simulink model "ProdSys_MakeToOrderPUSH_optionalWIPCap"  (R2015a)
settings: Solver=ode45  SolverMode=SingleTasking  StartTime=0.0  StopTime=10.0  RelTol=1e-3
undefined symbols (not defined in the file or in its folder): se_randomizeseeds
libraries: simeventslib x6, simulink x1
(part 2 of 2)

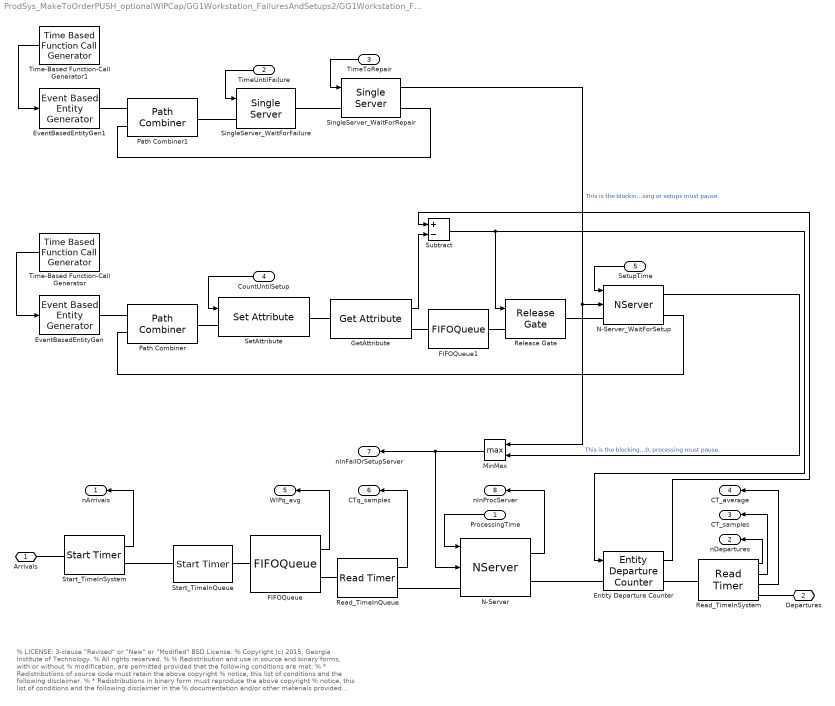
== system ProdSys_MakeToOrderPUSH_optionalWIPCap/GG1Workstation_FailuresAndSetups2/GG1Workstation_FailuresAndSetups ==
  note: % LICENSE: 3-clause "Revised" or "New" or "Modified" BSD License.
      | % Copyright (c) 2015, Georgia Institute of Technology.
      | % All rights reserved.
      | %
      | % Redistribution and use in source and binary forms, with or without
      | % modification, are permitted provided that the following conditions are met:
      | % * Redistributions of source code must retain the above copyright
      | % notice, this list of conditions and the following disclaimer.
      | % * Redistributions in binary form must reproduce the above copyright
      | % notice, this list of conditions and the following disclaimer in the
      | % documentation and/or other materials provided with the distribution.
      | % * Neither the name of the Georgia Institute of Technology nor the
      | % names of its contributors may be used to endorse or promote products
      | % derived from this software without specific prior written permission.
      | %
      | % THIS SOFTWARE IS PROVIDED BY THE COPYRIGHT HOLDERS AND CONTRIBUTORS "AS IS" AND
      | % ANY EXPRESS OR IMPLIED WARRANTIES, INCLUDING, BUT NOT LIMITED TO, THE IMPLIED
      | % WARRANTIES OF MERCHANTABILITY AND FITNESS FOR A PARTICULAR PURPOSE ARE
      | % DISCLAIMED. IN NO EVENT SHALL THE GEORGIA INSTITUTE OF TECHNOLOGY BE LIABLE FOR
      | % ANY DIRECT, INDIRECT, INCIDENTAL, SPECIAL, EXEMPLARY, OR CONSEQUENTIAL DAMAGES
      | % (INCLUDING, BUT NOT LIMITED TO, PROCUREMENT OF SUBSTITUTE GOODS OR SERVICES;
      | % LOSS OF USE, DATA, OR PROFITS; OR BUSINESS INTERRUPTION) HOWEVER CAUSED AND
      | % ON ANY THEORY OF LIABILITY, WHETHER IN CONTRACT, STRICT LIABILITY, OR TORT
      | % (INCLUDING NEGLIGENCE OR OTHERWISE) ARISING IN ANY WAY OUT OF THE USE OF THIS
      | % SOFTWARE, EVEN IF ADVISED OF THE POSSIBILITY OF SUCH DAMAGE.
  ProcessingTime : Inport
  TimeUntilFailure : Inport  Port=2
  TimeToRepair : Inport  Port=3
  CountUntilSetup : Inport  Port=4
  SetupTime : Inport  Port=5
  Entity Departure Counter : EntityDepartureCounter  NumberDepartedToSignal=on  NumberDepartedToAttribute=off  CounterResetTypeOption=Trigger from port tr
  EventBasedEntityGen : EventBasedEntityGenerator  GenerateEntitiesUpon=Function call from port fcn
  EventBasedEntityGen1 : EventBasedEntityGenerator  GenerateEntitiesUpon=Function call from port fcn
  FIFOQueue : FIFOQueue  Capacity=Capacity  StatAverageQueueLength=on
      settings: OutputPortMap=o3
  FIFOQueue1 : FIFOQueue  Capacity=Inf
  GetAttribute : GetAttribute  AttributeName=CountUntilSetup  EvaluatedDefaultAttributeValue={ []}
      settings: OutputPortMap=o1
  MinMax : MinMax  Function=max  Inputs=2
  N-Server : NServer  NumberOfServers=1  ServiceTimeFrom=Signal port t  AllowServiceControl=on  BlockWhileSignalOn=on  StatNumberInBlock=on
      settings: InputPortMap=u0,u1  OutputPortMap=o1
  N-Server_WaitForSetup : NServer  NumberOfServers=1  ServiceTimeFrom=Signal port t  AllowServiceControl=on  BlockWhileSignalOn=on  StatNumberInBlock=on
      settings: InputPortMap=u0,u1  OutputPortMap=o1
  Path Combiner : PathCombiner  NumberInputPorts=2
  Path Combiner1 : PathCombiner  NumberInputPorts=2
  Read_TimeInQueue : ReadTimer  TimerTag=TimeInQueue  StatTimeElapsed=on
      settings: OutputPortMap=o2
  Read_TimeInSystem : ReadTimer  TimerTag=TimeInSystem  StatNumberDeparted=on  StatTimeElapsed=on  StatAverageTimeElapsed=on
      settings: OutputPortMap=o0,o2,o3
  Release Gate : ReleaseGate  OpenGateUpon=Trigger from port tr
  SetAttribute : SetAttribute  AttributeName=CountUntilSetup  AttributeFrom=Signal port  EvaluatedAttributeValue={ []}
  SingleServer_WaitForFailure : SingleServer  ServiceTimeFrom=Signal port t  AttributeName=TimeUntilFailure
  SingleServer_WaitForRepair : SingleServer  ServiceTimeFrom=Signal port t  AttributeName=TimeToRepair  StatNumberInBlock=on
      settings: OutputPortMap=o1
  Start_TimeInQueue : StartTimer  TimerTag=TimeInQueue  TimerStartedOption=Restart
  Start_TimeInSystem : StartTimer  TimerTag=TimeInSystem  TimerStartedOption=Restart  StatNumberDeparted=on
  Subtract : Sum  Inputs=+-
  Time-Based Function-Call Generator : TimeBasedFunctionCallGenerator  EventGenerationMode=Only at simulation start
  Time-Based Function-Call Generator1 : TimeBasedFunctionCallGenerator  EventGenerationMode=Only at simulation start
  Arrivals : PMIOPort  Port=1  Side=Left
  Departures : PMIOPort  Port=2  Side=Right
  nArrivals : Outport
  nDepartures : Outport  Port=2
  CT_samples : Outport  Port=3
  CT_average : Outport  Port=4
  WIPq_avg : Outport  Port=5
  CTq_samples : Outport  Port=6
  nInFailOrSetupServer : Outport  Port=7
  nInProcServer : Outport  Port=8
  wires:
  MinMax/1 -> N-Server/2, nInFailOrSetupServer/1
  N-Server_WaitForSetup/1 -> MinMax/2  "This is the blocking signal from setups.  When >0, processing must pause."
  SingleServer_WaitForRepair/1 -> N-Server_WaitForSetup/2, MinMax/1  "This is the blocking signal from failures. When >0, processing or setups must pause."
  TimeUntilFailure/1 -> SingleServer_WaitForFailure/1
  TimeToRepair/1 -> SingleServer_WaitForRepair/1
  Time-Based Function-Call Generator1/1 -> EventBasedEntityGen1/1
  SetupTime/1 -> N-Server_WaitForSetup/1
  N-Server/1 -> nInProcServer/1
  Entity Departure Counter/1 -> Subtract/1
  GetAttribute/1 -> Subtract/2
  Subtract/1 -> Entity Departure Counter/1, Release Gate/1
  CountUntilSetup/1 -> SetAttribute/1
  Time-Based Function-Call Generator/1 -> EventBasedEntityGen/1
  Read_TimeInSystem/3 -> CT_average/1
  ProcessingTime/1 -> N-Server/1
  Read_TimeInSystem/1 -> nDepartures/1
  Start_TimeInSystem/1 -> nArrivals/1
  FIFOQueue/1 -> WIPq_avg/1
  Read_TimeInQueue/1 -> CTq_samples/1
  Read_TimeInSystem/2 -> CT_samples/1
  connections:
  Path Combiner1/RConn1 -- SingleServer_WaitForFailure/LConn1
  EventBasedEntityGen1/RConn1 -- Path Combiner1/LConn1
  SingleServer_WaitForRepair/LConn1 -- SingleServer_WaitForFailure/RConn1
  Path Combiner1/LConn2 -- SingleServer_WaitForRepair/RConn1
  SetAttribute/RConn1 -- GetAttribute/LConn1
  FIFOQueue1/RConn1 -- Release Gate/LConn1
  N-Server_WaitForSetup/LConn1 -- Release Gate/RConn1
  FIFOQueue1/LConn1 -- GetAttribute/RConn1
  Entity Departure Counter/RConn1 -- Read_TimeInSystem/LConn1
  N-Server/RConn1 -- Entity Departure Counter/LConn1
  Path Combiner/LConn2 -- N-Server_WaitForSetup/RConn1
  EventBasedEntityGen/RConn1 -- Path Combiner/LConn1
  Path Combiner/RConn1 -- SetAttribute/LConn1
  Start_TimeInQueue/RConn1 -- FIFOQueue/LConn1
  Read_TimeInQueue/RConn1 -- N-Server/LConn1
  Read_TimeInSystem/RConn1 -- Departures/RConn1
  Start_TimeInSystem/RConn1 -- Start_TimeInQueue/LConn1
  FIFOQueue/RConn1 -- Read_TimeInQueue/LConn1
  Arrivals/RConn1 -- Start_TimeInSystem/LConn1

== system ProdSys_MakeToOrderPUSH_optionalWIPCap/GG1Workstation_FailuresAndSetups3/ComputeTH ==
  CurrentTime : Inport
  nDepartures : Inport  Port=2
  Derivative : Derivative
  Divide1 : Product  Inputs=/*
  Event to Timed Signal1 : EventToTimedSignal
  TH_average : Outport
  TH_samples : Outport  Port=2
  wires:
  nDepartures/1 -> Event to Timed Signal1/1
  Derivative/1 -> TH_samples/1
  Divide1/1 -> TH_average/1
  Event to Timed Signal1/1 -> Divide1/2, Derivative/1
  CurrentTime/1 -> Divide1/1

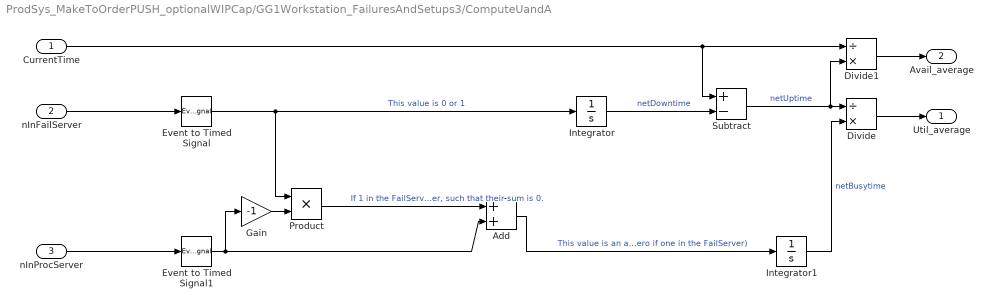
== system ProdSys_MakeToOrderPUSH_optionalWIPCap/GG1Workstation_FailuresAndSetups3/ComputeUandA ==
  CurrentTime : Inport
  nInFailServer : Inport  Port=2
  nInProcServer : Inport  Port=3
  Add : Sum
  Divide : Product  Inputs=/*
  Divide1 : Product  Inputs=/*
  Event to Timed Signal : EventToTimedSignal
  Event to Timed Signal1 : EventToTimedSignal
  Gain : Gain  Gain=-1
  Integrator : Integrator
  Integrator1 : Integrator
  Product : Product
  Subtract : Sum  Inputs=+-
  Util_average : Outport
  Avail_average : Outport  Port=2
  wires:
  Divide1/1 -> Avail_average/1
  Event to Timed Signal1/1 -> Gain/1, Add/2
  Add/1 -> Integrator1/1  "This value is an adjusted number in the ProcServer (zero if one in the FailServer)"
  Product/1 -> Add/1  "If 1 in the FailServer, then this value should be negative the number in the ProcServer, such that their sum is 0."
  Gain/1 -> Product/2
  Integrator1/1 -> Divide/2  "netBusytime"
  Subtract/1 -> Divide1/2, Divide/1  "netUptime"
  Divide/1 -> Util_average/1
  CurrentTime/1 -> Divide1/1, Subtract/1
  Integrator/1 -> Subtract/2  "netDowntime"
  nInProcServer/1 -> Event to Timed Signal1/1
  nInFailServer/1 -> Event to Timed Signal/1
  Event to Timed Signal/1 -> Product/1, Integrator/1  "This value is 0 or 1"

== system ProdSys_MakeToOrderPUSH_optionalWIPCap/GG1Workstation_FailuresAndSetups3/ComputeWIP ==
  nArrivals : Inport
  nDepartures : Inport  Port=2
  CurrentTime : Inport  Port=3
  Divide : Product  Inputs=*/
  Event to Timed Signal : EventToTimedSignal
  Integrator : Integrator
  Subtract : Sum  Inputs=+-
  WIP_samples : Outport
  WIP_average : Outport  Port=2
  wires:
  CurrentTime/1 -> Divide/2
  nDepartures/1 -> Subtract/2
  nArrivals/1 -> Subtract/1
  Integrator/1 -> Divide/1
  Divide/1 -> WIP_average/1
  Event to Timed Signal/1 -> Integrator/1
  Subtract/1 -> Event to Timed Signal/1, WIP_samples/1

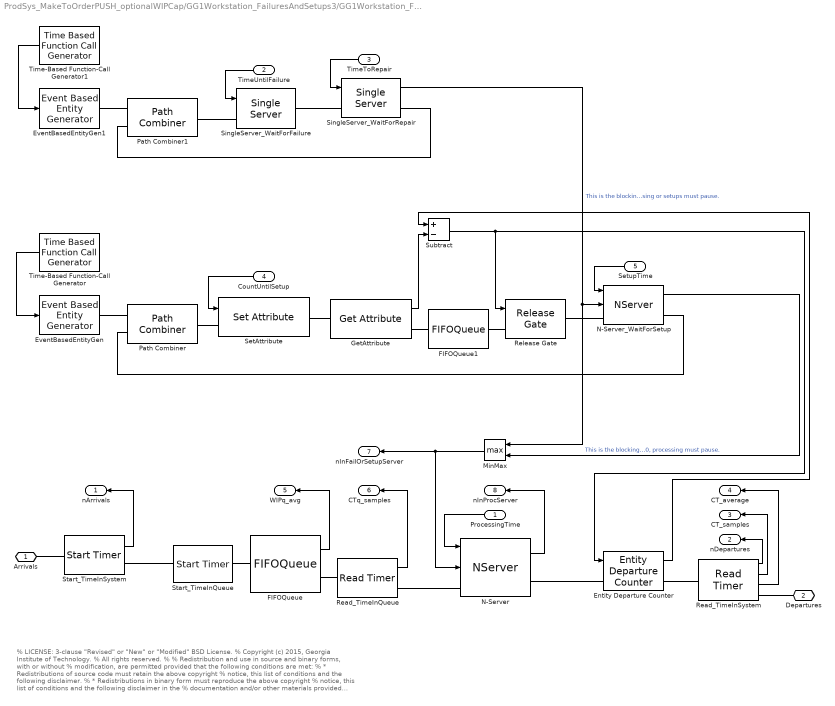
== system ProdSys_MakeToOrderPUSH_optionalWIPCap/GG1Workstation_FailuresAndSetups3/GG1Workstation_FailuresAndSetups ==
  note: % LICENSE: 3-clause "Revised" or "New" or "Modified" BSD License.
      | % Copyright (c) 2015, Georgia Institute of Technology.
      | % All rights reserved.
      | %
      | % Redistribution and use in source and binary forms, with or without
      | % modification, are permitted provided that the following conditions are met:
      | % * Redistributions of source code must retain the above copyright
      | % notice, this list of conditions and the following disclaimer.
      | % * Redistributions in binary form must reproduce the above copyright
      | % notice, this list of conditions and the following disclaimer in the
      | % documentation and/or other materials provided with the distribution.
      | % * Neither the name of the Georgia Institute of Technology nor the
      | % names of its contributors may be used to endorse or promote products
      | % derived from this software without specific prior written permission.
      | %
      | % THIS SOFTWARE IS PROVIDED BY THE COPYRIGHT HOLDERS AND CONTRIBUTORS "AS IS" AND
      | % ANY EXPRESS OR IMPLIED WARRANTIES, INCLUDING, BUT NOT LIMITED TO, THE IMPLIED
      | % WARRANTIES OF MERCHANTABILITY AND FITNESS FOR A PARTICULAR PURPOSE ARE
      | % DISCLAIMED. IN NO EVENT SHALL THE GEORGIA INSTITUTE OF TECHNOLOGY BE LIABLE FOR
      | % ANY DIRECT, INDIRECT, INCIDENTAL, SPECIAL, EXEMPLARY, OR CONSEQUENTIAL DAMAGES
      | % (INCLUDING, BUT NOT LIMITED TO, PROCUREMENT OF SUBSTITUTE GOODS OR SERVICES;
      | % LOSS OF USE, DATA, OR PROFITS; OR BUSINESS INTERRUPTION) HOWEVER CAUSED AND
      | % ON ANY THEORY OF LIABILITY, WHETHER IN CONTRACT, STRICT LIABILITY, OR TORT
      | % (INCLUDING NEGLIGENCE OR OTHERWISE) ARISING IN ANY WAY OUT OF THE USE OF THIS
      | % SOFTWARE, EVEN IF ADVISED OF THE POSSIBILITY OF SUCH DAMAGE.
  ProcessingTime : Inport
  TimeUntilFailure : Inport  Port=2
  TimeToRepair : Inport  Port=3
  CountUntilSetup : Inport  Port=4
  SetupTime : Inport  Port=5
  Entity Departure Counter : EntityDepartureCounter  NumberDepartedToSignal=on  NumberDepartedToAttribute=off  CounterResetTypeOption=Trigger from port tr
  EventBasedEntityGen : EventBasedEntityGenerator  GenerateEntitiesUpon=Function call from port fcn
  EventBasedEntityGen1 : EventBasedEntityGenerator  GenerateEntitiesUpon=Function call from port fcn
  FIFOQueue : FIFOQueue  Capacity=Capacity  StatAverageQueueLength=on
      settings: OutputPortMap=o3
  FIFOQueue1 : FIFOQueue  Capacity=Inf
  GetAttribute : GetAttribute  AttributeName=CountUntilSetup  EvaluatedDefaultAttributeValue={ []}
      settings: OutputPortMap=o1
  MinMax : MinMax  Function=max  Inputs=2
  N-Server : NServer  NumberOfServers=1  ServiceTimeFrom=Signal port t  AllowServiceControl=on  BlockWhileSignalOn=on  StatNumberInBlock=on
      settings: InputPortMap=u0,u1  OutputPortMap=o1
  N-Server_WaitForSetup : NServer  NumberOfServers=1  ServiceTimeFrom=Signal port t  AllowServiceControl=on  BlockWhileSignalOn=on  StatNumberInBlock=on
      settings: InputPortMap=u0,u1  OutputPortMap=o1
  Path Combiner : PathCombiner  NumberInputPorts=2
  Path Combiner1 : PathCombiner  NumberInputPorts=2
  Read_TimeInQueue : ReadTimer  TimerTag=TimeInQueue  StatTimeElapsed=on
      settings: OutputPortMap=o2
  Read_TimeInSystem : ReadTimer  TimerTag=TimeInSystem  StatNumberDeparted=on  StatTimeElapsed=on  StatAverageTimeElapsed=on
      settings: OutputPortMap=o0,o2,o3
  Release Gate : ReleaseGate  OpenGateUpon=Trigger from port tr
  SetAttribute : SetAttribute  AttributeName=CountUntilSetup  AttributeFrom=Signal port  EvaluatedAttributeValue={ []}
  SingleServer_WaitForFailure : SingleServer  ServiceTimeFrom=Signal port t  AttributeName=TimeUntilFailure
  SingleServer_WaitForRepair : SingleServer  ServiceTimeFrom=Signal port t  AttributeName=TimeToRepair  StatNumberInBlock=on
      settings: OutputPortMap=o1
  Start_TimeInQueue : StartTimer  TimerTag=TimeInQueue  TimerStartedOption=Restart
  Start_TimeInSystem : StartTimer  TimerTag=TimeInSystem  TimerStartedOption=Restart  StatNumberDeparted=on
  Subtract : Sum  Inputs=+-
  Time-Based Function-Call Generator : TimeBasedFunctionCallGenerator  EventGenerationMode=Only at simulation start
  Time-Based Function-Call Generator1 : TimeBasedFunctionCallGenerator  EventGenerationMode=Only at simulation start
  Arrivals : PMIOPort  Port=1  Side=Left
  Departures : PMIOPort  Port=2  Side=Right
  nArrivals : Outport
  nDepartures : Outport  Port=2
  CT_samples : Outport  Port=3
  CT_average : Outport  Port=4
  WIPq_avg : Outport  Port=5
  CTq_samples : Outport  Port=6
  nInFailOrSetupServer : Outport  Port=7
  nInProcServer : Outport  Port=8
  wires:
  MinMax/1 -> N-Server/2, nInFailOrSetupServer/1
  N-Server_WaitForSetup/1 -> MinMax/2  "This is the blocking signal from setups.  When >0, processing must pause."
  SingleServer_WaitForRepair/1 -> N-Server_WaitForSetup/2, MinMax/1  "This is the blocking signal from failures. When >0, processing or setups must pause."
  TimeUntilFailure/1 -> SingleServer_WaitForFailure/1
  TimeToRepair/1 -> SingleServer_WaitForRepair/1
  Time-Based Function-Call Generator1/1 -> EventBasedEntityGen1/1
  SetupTime/1 -> N-Server_WaitForSetup/1
  N-Server/1 -> nInProcServer/1
  Entity Departure Counter/1 -> Subtract/1
  GetAttribute/1 -> Subtract/2
  Subtract/1 -> Entity Departure Counter/1, Release Gate/1
  CountUntilSetup/1 -> SetAttribute/1
  Time-Based Function-Call Generator/1 -> EventBasedEntityGen/1
  Read_TimeInSystem/3 -> CT_average/1
  ProcessingTime/1 -> N-Server/1
  Read_TimeInSystem/1 -> nDepartures/1
  Start_TimeInSystem/1 -> nArrivals/1
  FIFOQueue/1 -> WIPq_avg/1
  Read_TimeInQueue/1 -> CTq_samples/1
  Read_TimeInSystem/2 -> CT_samples/1
  connections:
  Path Combiner1/RConn1 -- SingleServer_WaitForFailure/LConn1
  EventBasedEntityGen1/RConn1 -- Path Combiner1/LConn1
  SingleServer_WaitForRepair/LConn1 -- SingleServer_WaitForFailure/RConn1
  Path Combiner1/LConn2 -- SingleServer_WaitForRepair/RConn1
  SetAttribute/RConn1 -- GetAttribute/LConn1
  FIFOQueue1/RConn1 -- Release Gate/LConn1
  N-Server_WaitForSetup/LConn1 -- Release Gate/RConn1
  FIFOQueue1/LConn1 -- GetAttribute/RConn1
  Entity Departure Counter/RConn1 -- Read_TimeInSystem/LConn1
  N-Server/RConn1 -- Entity Departure Counter/LConn1
  Path Combiner/LConn2 -- N-Server_WaitForSetup/RConn1
  EventBasedEntityGen/RConn1 -- Path Combiner/LConn1
  Path Combiner/RConn1 -- SetAttribute/LConn1
  Start_TimeInQueue/RConn1 -- FIFOQueue/LConn1
  Read_TimeInQueue/RConn1 -- N-Server/LConn1
  Read_TimeInSystem/RConn1 -- Departures/RConn1
  Start_TimeInSystem/RConn1 -- Start_TimeInQueue/LConn1
  FIFOQueue/RConn1 -- Read_TimeInQueue/LConn1
  Arrivals/RConn1 -- Start_TimeInSystem/LConn1

== system ProdSys_MakeToOrderPUSH_optionalWIPCap/GG1Workstation_FailuresAndSetups4/ComputeTH ==
  CurrentTime : Inport
  nDepartures : Inport  Port=2
  Derivative : Derivative
  Divide1 : Product  Inputs=/*
  Event to Timed Signal1 : EventToTimedSignal
  TH_average : Outport
  TH_samples : Outport  Port=2
  wires:
  nDepartures/1 -> Event to Timed Signal1/1
  Derivative/1 -> TH_samples/1
  Divide1/1 -> TH_average/1
  Event to Timed Signal1/1 -> Divide1/2, Derivative/1
  CurrentTime/1 -> Divide1/1

== system ProdSys_MakeToOrderPUSH_optionalWIPCap/GG1Workstation_FailuresAndSetups4/ComputeUandA ==
  CurrentTime : Inport
  nInFailServer : Inport  Port=2
  nInProcServer : Inport  Port=3
  Add : Sum
  Divide : Product  Inputs=/*
  Divide1 : Product  Inputs=/*
  Event to Timed Signal : EventToTimedSignal
  Event to Timed Signal1 : EventToTimedSignal
  Gain : Gain  Gain=-1
  Integrator : Integrator
  Integrator1 : Integrator
  Product : Product
  Subtract : Sum  Inputs=+-
  Util_average : Outport
  Avail_average : Outport  Port=2
  wires:
  Divide1/1 -> Avail_average/1
  Event to Timed Signal1/1 -> Gain/1, Add/2
  Add/1 -> Integrator1/1  "This value is an adjusted number in the ProcServer (zero if one in the FailServer)"
  Product/1 -> Add/1  "If 1 in the FailServer, then this value should be negative the number in the ProcServer, such that their sum is 0."
  Gain/1 -> Product/2
  Integrator1/1 -> Divide/2  "netBusytime"
  Subtract/1 -> Divide1/2, Divide/1  "netUptime"
  Divide/1 -> Util_average/1
  CurrentTime/1 -> Divide1/1, Subtract/1
  Integrator/1 -> Subtract/2  "netDowntime"
  nInProcServer/1 -> Event to Timed Signal1/1
  nInFailServer/1 -> Event to Timed Signal/1
  Event to Timed Signal/1 -> Product/1, Integrator/1  "This value is 0 or 1"

== system ProdSys_MakeToOrderPUSH_optionalWIPCap/GG1Workstation_FailuresAndSetups4/ComputeWIP ==
  nArrivals : Inport
  nDepartures : Inport  Port=2
  CurrentTime : Inport  Port=3
  Divide : Product  Inputs=*/
  Event to Timed Signal : EventToTimedSignal
  Integrator : Integrator
  Subtract : Sum  Inputs=+-
  WIP_samples : Outport
  WIP_average : Outport  Port=2
  wires:
  CurrentTime/1 -> Divide/2
  nDepartures/1 -> Subtract/2
  nArrivals/1 -> Subtract/1
  Integrator/1 -> Divide/1
  Divide/1 -> WIP_average/1
  Event to Timed Signal/1 -> Integrator/1
  Subtract/1 -> Event to Timed Signal/1, WIP_samples/1

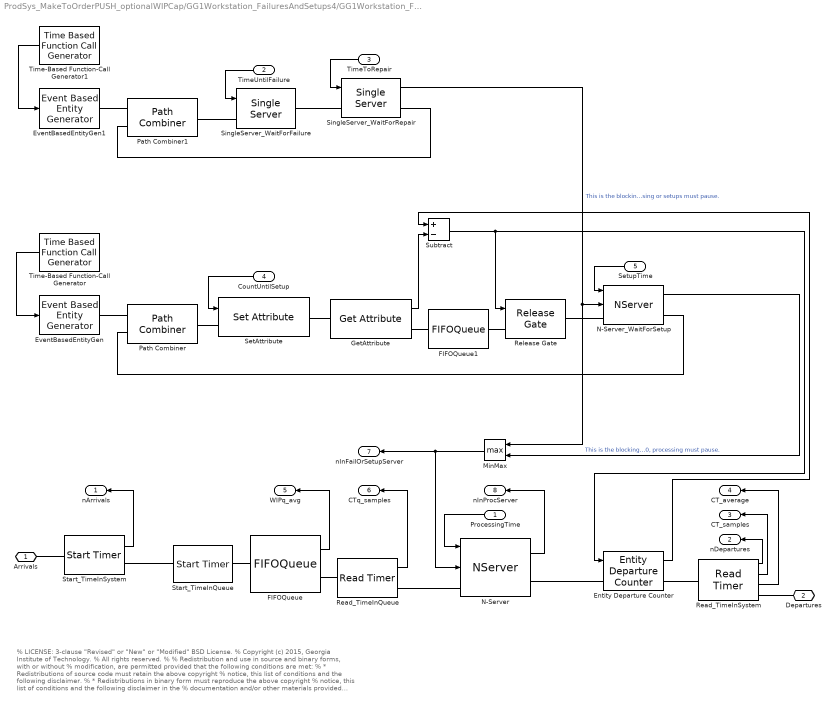
== system ProdSys_MakeToOrderPUSH_optionalWIPCap/GG1Workstation_FailuresAndSetups4/GG1Workstation_FailuresAndSetups ==
  note: % LICENSE: 3-clause "Revised" or "New" or "Modified" BSD License.
      | % Copyright (c) 2015, Georgia Institute of Technology.
      | % All rights reserved.
      | %
      | % Redistribution and use in source and binary forms, with or without
      | % modification, are permitted provided that the following conditions are met:
      | % * Redistributions of source code must retain the above copyright
      | % notice, this list of conditions and the following disclaimer.
      | % * Redistributions in binary form must reproduce the above copyright
      | % notice, this list of conditions and the following disclaimer in the
      | % documentation and/or other materials provided with the distribution.
      | % * Neither the name of the Georgia Institute of Technology nor the
      | % names of its contributors may be used to endorse or promote products
      | % derived from this software without specific prior written permission.
      | %
      | % THIS SOFTWARE IS PROVIDED BY THE COPYRIGHT HOLDERS AND CONTRIBUTORS "AS IS" AND
      | % ANY EXPRESS OR IMPLIED WARRANTIES, INCLUDING, BUT NOT LIMITED TO, THE IMPLIED
      | % WARRANTIES OF MERCHANTABILITY AND FITNESS FOR A PARTICULAR PURPOSE ARE
      | % DISCLAIMED. IN NO EVENT SHALL THE GEORGIA INSTITUTE OF TECHNOLOGY BE LIABLE FOR
      | % ANY DIRECT, INDIRECT, INCIDENTAL, SPECIAL, EXEMPLARY, OR CONSEQUENTIAL DAMAGES
      | % (INCLUDING, BUT NOT LIMITED TO, PROCUREMENT OF SUBSTITUTE GOODS OR SERVICES;
      | % LOSS OF USE, DATA, OR PROFITS; OR BUSINESS INTERRUPTION) HOWEVER CAUSED AND
      | % ON ANY THEORY OF LIABILITY, WHETHER IN CONTRACT, STRICT LIABILITY, OR TORT
      | % (INCLUDING NEGLIGENCE OR OTHERWISE) ARISING IN ANY WAY OUT OF THE USE OF THIS
      | % SOFTWARE, EVEN IF ADVISED OF THE POSSIBILITY OF SUCH DAMAGE.
  ProcessingTime : Inport
  TimeUntilFailure : Inport  Port=2
  TimeToRepair : Inport  Port=3
  CountUntilSetup : Inport  Port=4
  SetupTime : Inport  Port=5
  Entity Departure Counter : EntityDepartureCounter  NumberDepartedToSignal=on  NumberDepartedToAttribute=off  CounterResetTypeOption=Trigger from port tr
  EventBasedEntityGen : EventBasedEntityGenerator  GenerateEntitiesUpon=Function call from port fcn
  EventBasedEntityGen1 : EventBasedEntityGenerator  GenerateEntitiesUpon=Function call from port fcn
  FIFOQueue : FIFOQueue  Capacity=Capacity  StatAverageQueueLength=on
      settings: OutputPortMap=o3
  FIFOQueue1 : FIFOQueue  Capacity=Inf
  GetAttribute : GetAttribute  AttributeName=CountUntilSetup  EvaluatedDefaultAttributeValue={ []}
      settings: OutputPortMap=o1
  MinMax : MinMax  Function=max  Inputs=2
  N-Server : NServer  NumberOfServers=1  ServiceTimeFrom=Signal port t  AllowServiceControl=on  BlockWhileSignalOn=on  StatNumberInBlock=on
      settings: InputPortMap=u0,u1  OutputPortMap=o1
  N-Server_WaitForSetup : NServer  NumberOfServers=1  ServiceTimeFrom=Signal port t  AllowServiceControl=on  BlockWhileSignalOn=on  StatNumberInBlock=on
      settings: InputPortMap=u0,u1  OutputPortMap=o1
  Path Combiner : PathCombiner  NumberInputPorts=2
  Path Combiner1 : PathCombiner  NumberInputPorts=2
  Read_TimeInQueue : ReadTimer  TimerTag=TimeInQueue  StatTimeElapsed=on
      settings: OutputPortMap=o2
  Read_TimeInSystem : ReadTimer  TimerTag=TimeInSystem  StatNumberDeparted=on  StatTimeElapsed=on  StatAverageTimeElapsed=on
      settings: OutputPortMap=o0,o2,o3
  Release Gate : ReleaseGate  OpenGateUpon=Trigger from port tr
  SetAttribute : SetAttribute  AttributeName=CountUntilSetup  AttributeFrom=Signal port  EvaluatedAttributeValue={ []}
  SingleServer_WaitForFailure : SingleServer  ServiceTimeFrom=Signal port t  AttributeName=TimeUntilFailure
  SingleServer_WaitForRepair : SingleServer  ServiceTimeFrom=Signal port t  AttributeName=TimeToRepair  StatNumberInBlock=on
      settings: OutputPortMap=o1
  Start_TimeInQueue : StartTimer  TimerTag=TimeInQueue  TimerStartedOption=Restart
  Start_TimeInSystem : StartTimer  TimerTag=TimeInSystem  TimerStartedOption=Restart  StatNumberDeparted=on
  Subtract : Sum  Inputs=+-
  Time-Based Function-Call Generator : TimeBasedFunctionCallGenerator  EventGenerationMode=Only at simulation start
  Time-Based Function-Call Generator1 : TimeBasedFunctionCallGenerator  EventGenerationMode=Only at simulation start
  Arrivals : PMIOPort  Port=1  Side=Left
  Departures : PMIOPort  Port=2  Side=Right
  nArrivals : Outport
  nDepartures : Outport  Port=2
  CT_samples : Outport  Port=3
  CT_average : Outport  Port=4
  WIPq_avg : Outport  Port=5
  CTq_samples : Outport  Port=6
  nInFailOrSetupServer : Outport  Port=7
  nInProcServer : Outport  Port=8
  wires:
  MinMax/1 -> N-Server/2, nInFailOrSetupServer/1
  N-Server_WaitForSetup/1 -> MinMax/2  "This is the blocking signal from setups.  When >0, processing must pause."
  SingleServer_WaitForRepair/1 -> N-Server_WaitForSetup/2, MinMax/1  "This is the blocking signal from failures. When >0, processing or setups must pause."
  TimeUntilFailure/1 -> SingleServer_WaitForFailure/1
  TimeToRepair/1 -> SingleServer_WaitForRepair/1
  Time-Based Function-Call Generator1/1 -> EventBasedEntityGen1/1
  SetupTime/1 -> N-Server_WaitForSetup/1
  N-Server/1 -> nInProcServer/1
  Entity Departure Counter/1 -> Subtract/1
  GetAttribute/1 -> Subtract/2
  Subtract/1 -> Entity Departure Counter/1, Release Gate/1
  CountUntilSetup/1 -> SetAttribute/1
  Time-Based Function-Call Generator/1 -> EventBasedEntityGen/1
  Read_TimeInSystem/3 -> CT_average/1
  ProcessingTime/1 -> N-Server/1
  Read_TimeInSystem/1 -> nDepartures/1
  Start_TimeInSystem/1 -> nArrivals/1
  FIFOQueue/1 -> WIPq_avg/1
  Read_TimeInQueue/1 -> CTq_samples/1
  Read_TimeInSystem/2 -> CT_samples/1
  connections:
  Path Combiner1/RConn1 -- SingleServer_WaitForFailure/LConn1
  EventBasedEntityGen1/RConn1 -- Path Combiner1/LConn1
  SingleServer_WaitForRepair/LConn1 -- SingleServer_WaitForFailure/RConn1
  Path Combiner1/LConn2 -- SingleServer_WaitForRepair/RConn1
  SetAttribute/RConn1 -- GetAttribute/LConn1
  FIFOQueue1/RConn1 -- Release Gate/LConn1
  N-Server_WaitForSetup/LConn1 -- Release Gate/RConn1
  FIFOQueue1/LConn1 -- GetAttribute/RConn1
  Entity Departure Counter/RConn1 -- Read_TimeInSystem/LConn1
  N-Server/RConn1 -- Entity Departure Counter/LConn1
  Path Combiner/LConn2 -- N-Server_WaitForSetup/RConn1
  EventBasedEntityGen/RConn1 -- Path Combiner/LConn1
  Path Combiner/RConn1 -- SetAttribute/LConn1
  Start_TimeInQueue/RConn1 -- FIFOQueue/LConn1
  Read_TimeInQueue/RConn1 -- N-Server/LConn1
  Read_TimeInSystem/RConn1 -- Departures/RConn1
  Start_TimeInSystem/RConn1 -- Start_TimeInQueue/LConn1
  FIFOQueue/RConn1 -- Read_TimeInQueue/LConn1
  Arrivals/RConn1 -- Start_TimeInSystem/LConn1
